simulink model "SWC_SCP_type"  (R2021b)
settings: Solver=FixedStepDiscrete  StartTime=0.0  StopTime=10.0  FixedStep=0.005  RelTol=1e-3
libraries: scp x1
settings Model: DataDictionary=APPTypes.sldd  Creator=FVT23010  LastModifiedBy=FVT23010
settings DataIOCC: SaveFormat=StructureWithTime
settings OptimizationCC: DefaultParameterBehavior=Inlined  EnhancedBackFolding=on  PassReuseOutputArgsAs=Individual arguments  ZeroExternalMemoryAtStartup=off  ZeroInternalMemoryAtStartup=off  OptimizeBlockOrder=speed  DifferentSizesBufferReuse=on  OptimizationCustomize=off  EfficientTunableParamExpr=on
settings DebuggingCC: ParameterTunabilityLossMsg=error
settings ModelReferenceCC: ModelReferenceNumInstancesAllowed=Single
settings SFSimCC: MATLABDynamicMemAlloc=off
settings RTWCC: Description=AUTOSAR  SystemTargetFile=autosar.tlc  GenCodeOnly=on  TemplateMakefile=ert_default_tmf
settings CodeAppCC: ForceParamTrailComments=on  IgnoreCustomStorageClasses=off  OperatorAnnotations=on  SimulinkDataObjDesc=on  SFDataObjDesc=on  InsertBlockDesc=on
settings STFCustomTargetCC: TargetLangStandard=C99 (ISO)  MultiwordLength=256  ParMdlRefBuildCompliant=on  CompOptLevelCompliant=on  IncludeMdlTerminateFcn=off  CombineOutputUpdateFcns=on  SuppressErrorStatus=on  ERTCustomFileBanners=on  SupportNonFinite=off  SupportComplex=off  SupportContinuousTime=off  SupportNonInlinedSFcns=off  RemoveResetFunc=on  MATLABClassNameForMDSCustomization=Simulink.SoftwareTarget.ERTCustomization  AutosarCompliant=on  GRTInterface=off  UseToolchainInfoCompliant=on  LookupTableObjectStructAxisOrder=2,1,3,4,...  LUTObjectStructOrderEvenSpacing=Size,Table,Breakpoints  SystemTargetFile=autosar.tlc
settings ERTTargetCC: TargetLangStandard=C99 (ISO)  ConcurrentExecutionCompliant=off  IncludeMdlTerminateFcn=off  SuppressErrorStatus=on  SupportNonFinite=off  SupportComplex=off  ModelStepFunctionPrototypeControlCompliant=off  CPPClassGenCompliant=off  AutosarCompliant=on  LookupTableObjectStructAxisOrder=2,1,3,4,...  LUTObjectStructOrderEvenSpacing=Size,Table,Breakpoints  InlinedParameterPlacement=NonHierarchical  ERTCustomFileTemplate=example_file_process.tlc

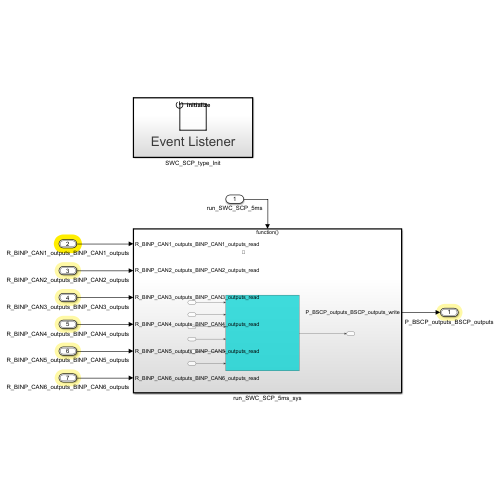
[thumbnail: Simulink's stored preview of the top-level diagram]
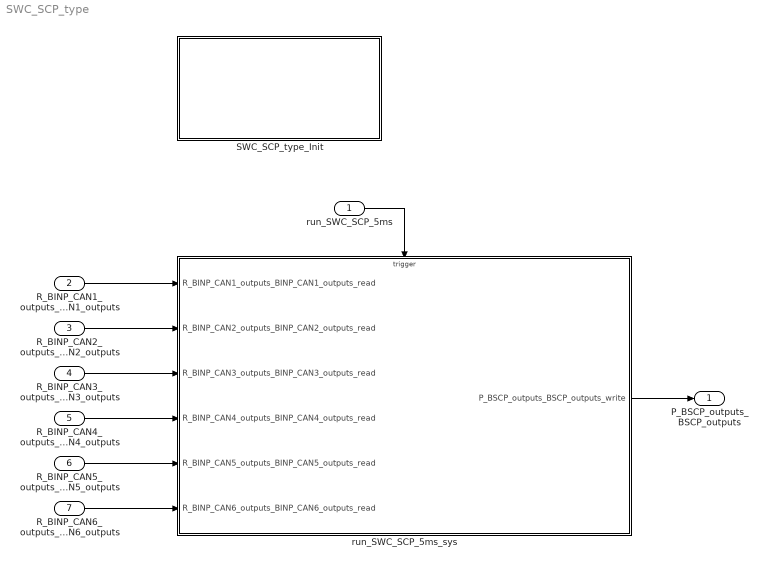
== system SWC_SCP_type ==
  run_SWC_SCP_5ms : Inport  SampleTime=0.005  OutputFunctionCall=on
  R_BINP_CAN1_outputs_BINP_CAN1_outputs : Inport  Port=2  OutDataTypeStr=Bus: BINP_CAN1_outputs  PortDimensions=1  BusOutputAsStruct=on
  R_BINP_CAN2_outputs_BINP_CAN2_outputs : Inport  Port=3  OutDataTypeStr=Bus: BINP_CAN2_outputs  PortDimensions=1  BusOutputAsStruct=on
  R_BINP_CAN3_outputs_BINP_CAN3_outputs : Inport  Port=4  OutDataTypeStr=Bus: BINP_CAN3_outputs  PortDimensions=1  BusOutputAsStruct=on
  R_BINP_CAN4_outputs_BINP_CAN4_outputs : Inport  Port=5  OutDataTypeStr=Bus: BINP_CAN4_outputs  PortDimensions=1  BusOutputAsStruct=on
  R_BINP_CAN5_outputs_BINP_CAN5_outputs : Inport  Port=6  OutDataTypeStr=Bus: BINP_CAN5_outputs  PortDimensions=1  BusOutputAsStruct=on
  R_BINP_CAN6_outputs_BINP_CAN6_outputs : Inport  Port=7  OutDataTypeStr=Bus: BINP_CAN6_outputs  PortDimensions=1  BusOutputAsStruct=on
  SWC_SCP_type_Init : Subsystem
  run_SWC_SCP_5ms_sys : Subsystem
  P_BSCP_outputs_BSCP_outputs : Outport  OutDataTypeStr=Bus: BSCP_outputs  PortDimensions=1  BusOutputAsStruct=on
  wires:
  R_BINP_CAN1_outputs_BINP_CAN1_outputs/1 -> run_SWC_SCP_5ms_sys/1(R_BINP_CAN1_outputs_BINP_CAN1_outputs_read)
  R_BINP_CAN2_outputs_BINP_CAN2_outputs/1 -> run_SWC_SCP_5ms_sys/2(R_BINP_CAN2_outputs_BINP_CAN2_outputs_read)
  R_BINP_CAN3_outputs_BINP_CAN3_outputs/1 -> run_SWC_SCP_5ms_sys/3(R_BINP_CAN3_outputs_BINP_CAN3_outputs_read)
  R_BINP_CAN4_outputs_BINP_CAN4_outputs/1 -> run_SWC_SCP_5ms_sys/4(R_BINP_CAN4_outputs_BINP_CAN4_outputs_read)
  R_BINP_CAN5_outputs_BINP_CAN5_outputs/1 -> run_SWC_SCP_5ms_sys/5(R_BINP_CAN5_outputs_BINP_CAN5_outputs_read)
  R_BINP_CAN6_outputs_BINP_CAN6_outputs/1 -> run_SWC_SCP_5ms_sys/6(R_BINP_CAN6_outputs_BINP_CAN6_outputs_read)
  run_SWC_SCP_5ms_sys/1(P_BSCP_outputs_BSCP_outputs_write) -> P_BSCP_outputs_BSCP_outputs/1
  run_SWC_SCP_5ms/1 -> run_SWC_SCP_5ms_sys/Trigger

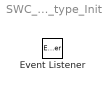
== system SWC_SCP_type/SWC_SCP_type_Init ==
  Event Listener : EventListener  EventName=reset

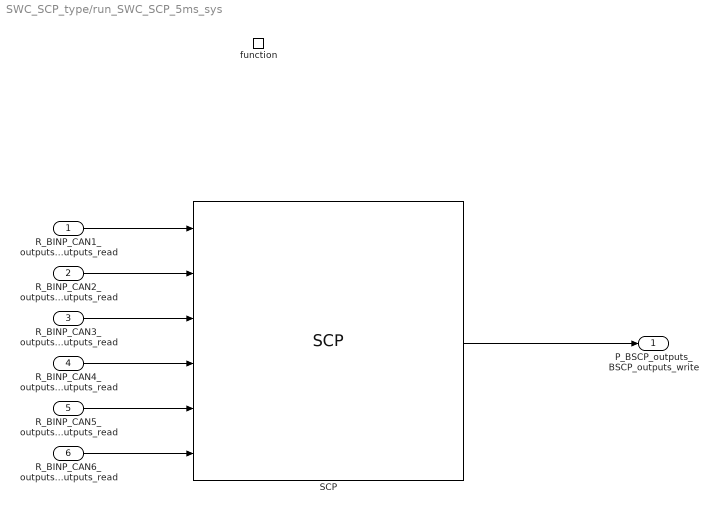
== system SWC_SCP_type/run_SWC_SCP_5ms_sys ==
  R_BINP_CAN1_outputs_BINP_CAN1_outputs_read : Inport
  R_BINP_CAN2_outputs_BINP_CAN2_outputs_read : Inport  Port=2
  R_BINP_CAN3_outputs_BINP_CAN3_outputs_read : Inport  Port=3
  R_BINP_CAN4_outputs_BINP_CAN4_outputs_read : Inport  Port=4
  R_BINP_CAN5_outputs_BINP_CAN5_outputs_read : Inport  Port=5
  R_BINP_CAN6_outputs_BINP_CAN6_outputs_read : Inport  Port=6
  function : TriggerPort  TriggerType=function-call  VariantControl=(inherit)  SampleTimeType=periodic  SampleTime=-1
  SCP : scp/SCP  SystemSampleTime=-1  VariantActivationTime=update diagram  Latency=0  AutoFrameSizeCalculation=off
  P_BSCP_outputs_BSCP_outputs_write : Outport
  wires:
  SCP/1 -> P_BSCP_outputs_BSCP_outputs_write/1
  R_BINP_CAN2_outputs_BINP_CAN2_outputs_read/1 -> SCP/2
  R_BINP_CAN1_outputs_BINP_CAN1_outputs_read/1 -> SCP/1
  R_BINP_CAN3_outputs_BINP_CAN3_outputs_read/1 -> SCP/3
  R_BINP_CAN4_outputs_BINP_CAN4_outputs_read/1 -> SCP/4
  R_BINP_CAN5_outputs_BINP_CAN5_outputs_read/1 -> SCP/5
  R_BINP_CAN6_outputs_BINP_CAN6_outputs_read/1 -> SCP/6
